simulink model "untitled3"  (R2025b)
settings: Solver=VariableStepAuto  StartTime=0.0  StopTime=10.0  RelTol=1e-3
undefined symbols (not defined in the file): bv, J, K, Kff, Km, Kp, L, R
libraries: slpidlib x8
settings Model: Creator=karadeli  LastModifiedBy=karadeli

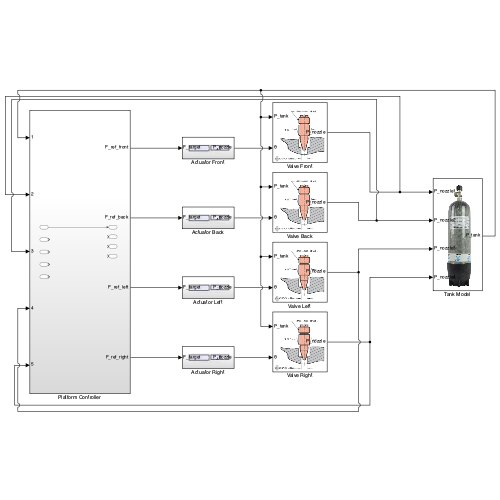
[thumbnail: Simulink's stored preview of the top-level diagram]
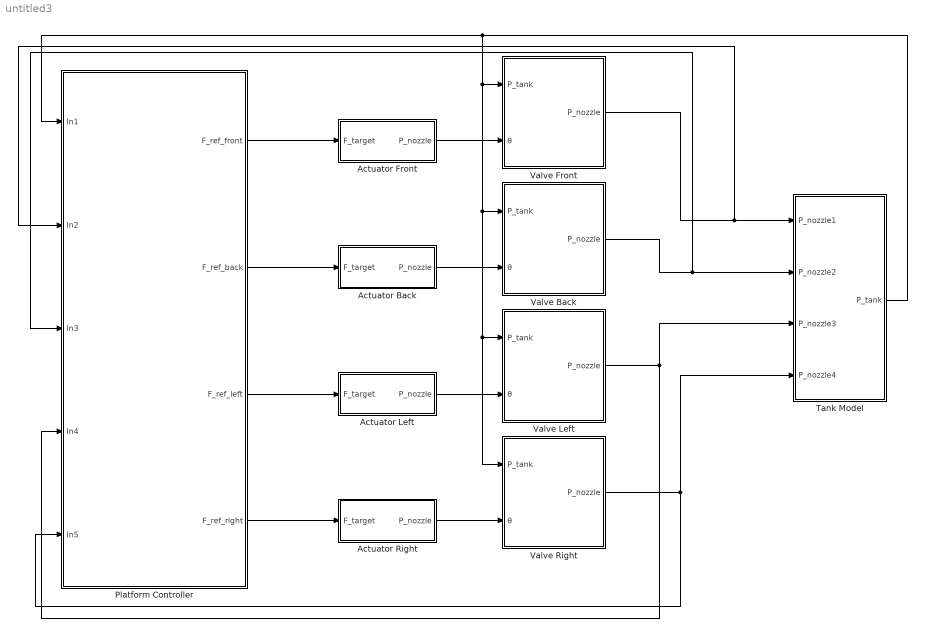
== system untitled3 ==
  Actuator Back : Subsystem
  Actuator Front : Subsystem
  Actuator Left : Subsystem
  Actuator Right : Subsystem
  Platform Controller : Subsystem
  Tank Model : Subsystem
      mask Display: image('Tank.png');
  Valve Back : Subsystem  mask{Parameter1=0}
      mask Display: image('Clippard-Needle-Valves-Overall.png');
  Valve Front : Subsystem  mask{Parameter1=0}
      mask Display: image('Clippard-Needle-Valves-Overall.png');
  Valve Left : Subsystem  mask{Parameter1=0}
      mask Display: image('Clippard-Needle-Valves-Overall.png');
  Valve Right : Subsystem  mask{Parameter1=0}
      mask Display: image('Clippard-Needle-Valves-Overall.png');
  wires:
  Platform Controller/1(F_ref_front) -> Actuator Front/1(F_target)
  Valve Front/1(P_nozzle) -> Platform Controller/2(In2), Tank Model/1(P_nozzle1)
  Tank Model/1(P_tank) -> Valve Right/1(P_tank), Valve Left/1(P_tank), Valve Back/1(P_tank), Valve Front/1(P_tank), Platform Controller/1(In1)
  Valve Back/1(P_nozzle) -> Tank Model/2(P_nozzle2), Platform Controller/3(In3)
  Valve Left/1(P_nozzle) -> Tank Model/3(P_nozzle3), Platform Controller/4(In4)
  Valve Right/1(P_nozzle) -> Tank Model/4(P_nozzle4), Platform Controller/5(In5)
  Actuator Front/1(P_nozzle) -> Valve Front/2(θ)
  Actuator Back/1(P_nozzle) -> Valve Back/2(θ)
  Actuator Left/1(P_nozzle) -> Valve Left/2(θ)
  Actuator Right/1(P_nozzle) -> Valve Right/2(θ)
  Platform Controller/2(F_ref_back) -> Actuator Back/1(F_target)
  Platform Controller/3(F_ref_left) -> Actuator Left/1(F_target)
  Platform Controller/4(F_ref_right) -> Actuator Right/1(F_target)

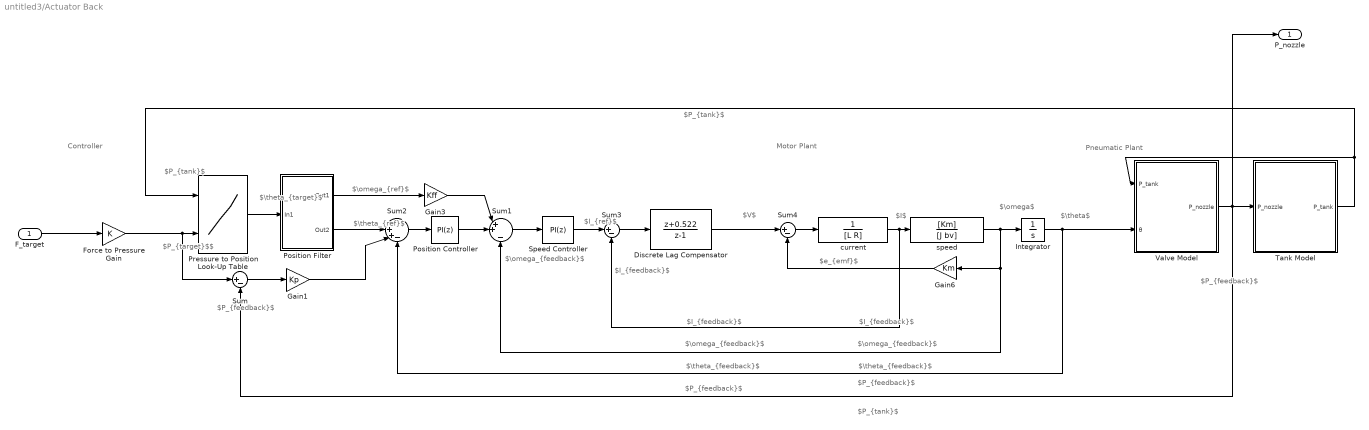
== system untitled3/Actuator Back ==
  note: $P_{tank}$
  note: $\theta_{target}$
  note: Pneumatic Plant
  note: $\theta_{ref}$
  note: $P_{feedback}$
  note: $I_{feedback}$
  note: $I_{ref}$
  note: $\theta_{feedback}$
  note: $e_{emf}$
  note: $P_{feedback}$
  note: $I_{feedback}$
  note: $P_{target}$$
  note: $\theta_{feedback}$
  note: Controller
  note: $P_{feedback}$
  note: $V$
  note: $\omega_{feedback}$
  note: $P_{tank}$
  note: $\omega_{feedback}$
  note: $\omega$
  note: $P_{feedback}$
  note: $I_{feedback}$
  note: $\omega_{feedback}$
  note: $\theta$
  note: Motor Plant
  note: $I$
  note: $P_{tank}$
  note: $\omega_{ref}$
  F_target : Inport
  Discrete Lag Compensator : DiscreteTransferFcn  Numerator=[1 0.522]  Denominator=[1 -1]
  Force to Pressure Gain : Gain  Gain=K
  Gain1 : Gain  Gain=Kp
  Gain3 : Gain  Gain=Kff
  Gain6 : Gain  Gain=Km
  Integrator : Integrator
  Position Controller : slpidlib/PID Controller  Controller=PI  Form=Parallel  TimeDomain=Discrete-time  UseExternalTs=off  SampleTime=-1  IntegratorMethod=Forward Euler  FilterMethod=Forward Euler  ControllerParametersSource=internal  P=1  I=1  UseKiTs=off  D=0  UseExternalDerivativeSource=off  N=100  UseFilter=on  TunerSelectOption=Transfer Function Based (PID Tuner App)  InitialConditionSource=internal  InitialConditionForIntegrator=0  InitialConditionForFilter=0  DifferentiatorICPrevScaledInput=0  ExternalReset=none  TrackingMode=off  Kt=1  LimitOutput=off  SatLimitsSource=internal  UpperSaturationLimit=inf  LowerSaturationLimit=-inf  LinearizeAsGain=on  AntiWindupMode=none  Kb=1  LimitIntegrator=off  UpperIntegratorSaturationLimit=inf  LowerIntegratorSaturationLimit=-inf  POutMin=[]  POutMax=[]  IOutMin=[]  IOutMax=[]  DOutMin=[]  DOutMax=[]  NOutMin=[]  NOutMax=[]  SumOutMin=[]  SumOutMax=[]  SaturationOutMin=[]  SaturationOutMax=[]  PParamMin=[]  PParamMax=[]  IParamMin=[]  IParamMax=[]  DParamMin=[]  DParamMax=[]  NParamMin=[]  NParamMax=[]  KbParamMin=[]  KbParamMax=[]  KtParamMin=[]  KtParamMax=[]  KbOutMin=[]  KbOutMax=[]  KtOutMin=[]  KtOutMax=[]  IntegratorOutMin=[]  IntegratorOutMax=[]  FilterOutMin=[]  FilterOutMax=[]  SumI1OutMin=[]  SumI1OutMax=[]  SumI2OutMin=[]  SumI2OutMax=[]  SumI3OutMin=[]  SumI3OutMax=[]  SumI4OutMin=[]  SumI4OutMax=[]  SumDOutMin=[]  SumDOutMax=[]  DifferentiatorOutMin=[]  DifferentiatorOutMax=[]  FilterDiffOutCoefMin=[]  FilterDiffOutCoefMax=[]  ReciprocalOutMin=[]  ReciprocalOutMax=[]  SumDenOutMin=[]  SumDenOutMax=[]  SumNumOutMin=[]  SumNumOutMax=[]  DivideOutMin=[]  DivideOutMax=[]  UdiffTsProdOutMin=[]  UdiffTsProdOutMax=[]  NTsProdOutMin=[]  NTsProdOutMax=[]  UintegralTsProdOutMin=[]  UintegralTsProdOutMax=[]  UngainTsProdOutMin=[]  UngainTsProdOutMax=[]  ClampingZeroOutDataTypeStr=Inherit: Inherit via back propagation  ClampingZeroOutMin=[]  ClampingZeroOutMax=[]  FilterDenConstantOutDataTypeStr=Inherit: Inherit via back propagation  FilterDenConstantOutMin=[]  FilterDenConstantOutMax=[]  PCopyOutDataTypeStr=Inherit: Inherit via back propagation  PCopyOutMin=[]  PCopyOutMax=[]  NCopyOutDataTypeStr=Inherit: Inherit via back propagation  NCopyOutMin=[]  NCopyOutMax=[]  IntegratorContinuousStateAttributes=''  IntegratorStateMustResolveToSignalObject=off  IntegratorRTWStateStorageClass=Auto  FilterContinuousStateAttributes=''  FilterStateMustResolveToSignalObject=off  FilterRTWStateStorageClass=Auto  ParallelPVariant=InternalParameters  IdealPVariant=Disabled  IVariant=InternalParameters  DVariant=Disabled  IntegratorVariant=Discrete  SatVariant=Disabled  AWVariant=Passthrough  PCopyVariant=Disabled  TRVariant=Disabled  FdbkBlocksVariant=Forward  IdealPFdbkVariant=Disabled  SatFdbkVariant=Disabled  DerivativeFilterVariant=Disabled  NVariant=Disabled  NCopyVariant=Disabled_SignalSpec  FilterICVariant=Disabled  IntegratorICVariant=InternalICs  ExternalResetVariant=Disabled  TRSumVariant=Passthrough  SumFdbkVariant=Disabled  SumVariant=Sum_PI  TsampFilterVariant=InternalTs  TsampNgainVariant=Passthrough  TsampIntegralVariant=Disabled_SignalSpec  ExternalSaturationOutDataTypeStr=Inherit: Same as second input  DerivativeSourceVariant=Disabled  PreIntVariant=InternalPreInt
  Position Filter : Subsystem
      mask Display: dpoly([1], [1/50 1], 's');
  Pressure to Position Look-Up Table : Lookup_n-D  BreakpointsForDimension1=[1:3]  BreakpointsForDimension2=[1:3]  InternalRulePriority=Speed  RndMeth=Simplest
      settings: InputPortMap=u0,u1
  Speed Controller : slpidlib/PID Controller  Controller=PI  Form=Parallel  TimeDomain=Discrete-time  UseExternalTs=off  SampleTime=-1  IntegratorMethod=Forward Euler  FilterMethod=Forward Euler  ControllerParametersSource=internal  P=1  I=1  UseKiTs=off  D=0  UseExternalDerivativeSource=off  N=100  UseFilter=on  TunerSelectOption=Transfer Function Based (PID Tuner App)  InitialConditionSource=internal  InitialConditionForIntegrator=0  InitialConditionForFilter=0  DifferentiatorICPrevScaledInput=0  ExternalReset=none  TrackingMode=off  Kt=1  LimitOutput=off  SatLimitsSource=internal  UpperSaturationLimit=inf  LowerSaturationLimit=-inf  LinearizeAsGain=on  AntiWindupMode=none  Kb=1  LimitIntegrator=off  UpperIntegratorSaturationLimit=inf  LowerIntegratorSaturationLimit=-inf  POutMin=[]  POutMax=[]  IOutMin=[]  IOutMax=[]  DOutMin=[]  DOutMax=[]  NOutMin=[]  NOutMax=[]  SumOutMin=[]  SumOutMax=[]  SaturationOutMin=[]  SaturationOutMax=[]  PParamMin=[]  PParamMax=[]  IParamMin=[]  IParamMax=[]  DParamMin=[]  DParamMax=[]  NParamMin=[]  NParamMax=[]  KbParamMin=[]  KbParamMax=[]  KtParamMin=[]  KtParamMax=[]  KbOutMin=[]  KbOutMax=[]  KtOutMin=[]  KtOutMax=[]  IntegratorOutMin=[]  IntegratorOutMax=[]  FilterOutMin=[]  FilterOutMax=[]  SumI1OutMin=[]  SumI1OutMax=[]  SumI2OutMin=[]  SumI2OutMax=[]  SumI3OutMin=[]  SumI3OutMax=[]  SumI4OutMin=[]  SumI4OutMax=[]  SumDOutMin=[]  SumDOutMax=[]  DifferentiatorOutMin=[]  DifferentiatorOutMax=[]  FilterDiffOutCoefMin=[]  FilterDiffOutCoefMax=[]  ReciprocalOutMin=[]  ReciprocalOutMax=[]  SumDenOutMin=[]  SumDenOutMax=[]  SumNumOutMin=[]  SumNumOutMax=[]  DivideOutMin=[]  DivideOutMax=[]  UdiffTsProdOutMin=[]  UdiffTsProdOutMax=[]  NTsProdOutMin=[]  NTsProdOutMax=[]  UintegralTsProdOutMin=[]  UintegralTsProdOutMax=[]  UngainTsProdOutMin=[]  UngainTsProdOutMax=[]  ClampingZeroOutDataTypeStr=Inherit: Inherit via back propagation  ClampingZeroOutMin=[]  ClampingZeroOutMax=[]  FilterDenConstantOutDataTypeStr=Inherit: Inherit via back propagation  FilterDenConstantOutMin=[]  FilterDenConstantOutMax=[]  PCopyOutDataTypeStr=Inherit: Inherit via back propagation  PCopyOutMin=[]  PCopyOutMax=[]  NCopyOutDataTypeStr=Inherit: Inherit via back propagation  NCopyOutMin=[]  NCopyOutMax=[]  IntegratorContinuousStateAttributes=''  IntegratorStateMustResolveToSignalObject=off  IntegratorRTWStateStorageClass=Auto  FilterContinuousStateAttributes=''  FilterStateMustResolveToSignalObject=off  FilterRTWStateStorageClass=Auto  ParallelPVariant=InternalParameters  IdealPVariant=Disabled  IVariant=InternalParameters  DVariant=Disabled  IntegratorVariant=Discrete  SatVariant=Disabled  AWVariant=Passthrough  PCopyVariant=Disabled  TRVariant=Disabled  FdbkBlocksVariant=Forward  IdealPFdbkVariant=Disabled  SatFdbkVariant=Disabled  DerivativeFilterVariant=Disabled  NVariant=Disabled  NCopyVariant=Disabled_SignalSpec  FilterICVariant=Disabled  IntegratorICVariant=InternalICs  ExternalResetVariant=Disabled  TRSumVariant=Passthrough  SumFdbkVariant=Disabled  SumVariant=Sum_PI  TsampFilterVariant=InternalTs  TsampNgainVariant=Passthrough  TsampIntegralVariant=Disabled_SignalSpec  ExternalSaturationOutDataTypeStr=Inherit: Same as second input  DerivativeSourceVariant=Disabled  PreIntVariant=InternalPreInt
  Sum : Sum  Inputs=|+-
  Sum1 : Sum  Inputs=|++|-
  Sum2 : Sum  Inputs=||++-
  Sum3 : Sum  Inputs=|+-
  Sum4 : Sum  Inputs=|+-
  Tank Model : Subsystem
      mask Display: image('Tank.png');
  Valve Model : Subsystem  mask{Parameter1=0}
      mask Display: image('Clippard-Needle-Valves-Overall.png');
  current : TransferFcn  Denominator=[L R]  ContinuousStateAttributes='current'
  speed : TransferFcn  Numerator=[Km]  Denominator=[J bv]  ContinuousStateAttributes='speed'
  P_nozzle : Outport
  wires:
  speed/1 -> Sum1/3, Gain6/1, Integrator/1
  Tank Model/1(P_tank) -> Pressure to Position Look-Up Table/1, Valve Model/1(P_tank)
  Position Controller/1 -> Sum1/2
  Sum/1 -> Gain1/1
  Pressure to Position Look-Up Table/1 -> Position Filter/1(In1)
  Force to Pressure Gain/1 -> Pressure to Position Look-Up Table/2, Sum/1
  Gain3/1 -> Sum1/1
  F_target/1 -> Force to Pressure Gain/1
  Position Filter/1(Out1) -> Gain3/1
  Sum4/1 -> current/1
  Sum2/1 -> Position Controller/1
  Valve Model/1(P_nozzle) -> Tank Model/1(P_nozzle), P_nozzle/1, Sum/2
  Gain6/1 -> Sum4/2
  Discrete Lag Compensator/1 -> Sum4/1
  Sum3/1 -> Discrete Lag Compensator/1
  Position Filter/2(Out2) -> Sum2/1
  current/1 -> speed/1, Sum3/2
  Speed Controller/1 -> Sum3/1
  Sum1/1 -> Speed Controller/1
  Integrator/1 -> Sum2/3, Valve Model/2(θ)
  Gain1/1 -> Sum2/2

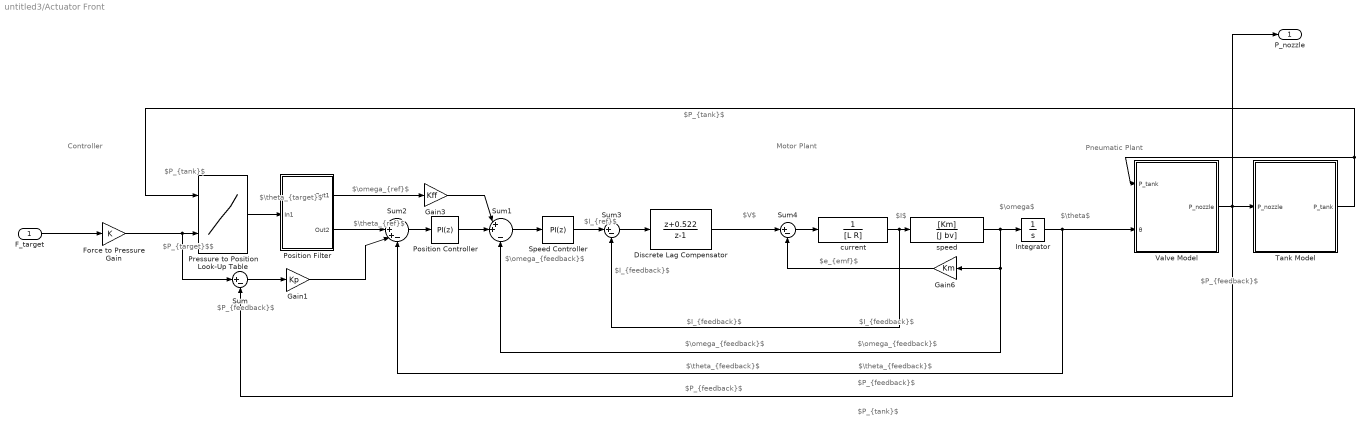
== system untitled3/Actuator Front ==
  note: $\omega_{ref}$
  note: $P_{tank}$
  note: $I$
  note: Motor Plant
  note: $\theta$
  note: $\omega_{feedback}$
  note: $I_{feedback}$
  note: $P_{feedback}$
  note: $\omega$
  note: $\omega_{feedback}$
  note: $P_{tank}$
  note: $\omega_{feedback}$
  note: $V$
  note: $P_{feedback}$
  note: Controller
  note: $\theta_{feedback}$
  note: $P_{target}$$
  note: $I_{feedback}$
  note: $P_{feedback}$
  note: $e_{emf}$
  note: $\theta_{feedback}$
  note: $I_{ref}$
  note: $I_{feedback}$
  note: $P_{feedback}$
  note: $\theta_{ref}$
  note: Pneumatic Plant
  note: $\theta_{target}$
  note: $P_{tank}$
  F_target : Inport
  Discrete Lag Compensator : DiscreteTransferFcn  Numerator=[1 0.522]  Denominator=[1 -1]
  Force to Pressure Gain : Gain  Gain=K
  Gain1 : Gain  Gain=Kp
  Gain3 : Gain  Gain=Kff
  Gain6 : Gain  Gain=Km
  Integrator : Integrator
  Position Controller : slpidlib/PID Controller  Controller=PI  Form=Parallel  TimeDomain=Discrete-time  UseExternalTs=off  SampleTime=-1  IntegratorMethod=Forward Euler  FilterMethod=Forward Euler  ControllerParametersSource=internal  P=1  I=1  UseKiTs=off  D=0  UseExternalDerivativeSource=off  N=100  UseFilter=on  TunerSelectOption=Transfer Function Based (PID Tuner App)  InitialConditionSource=internal  InitialConditionForIntegrator=0  InitialConditionForFilter=0  DifferentiatorICPrevScaledInput=0  ExternalReset=none  TrackingMode=off  Kt=1  LimitOutput=off  SatLimitsSource=internal  UpperSaturationLimit=inf  LowerSaturationLimit=-inf  LinearizeAsGain=on  AntiWindupMode=none  Kb=1  LimitIntegrator=off  UpperIntegratorSaturationLimit=inf  LowerIntegratorSaturationLimit=-inf  POutMin=[]  POutMax=[]  IOutMin=[]  IOutMax=[]  DOutMin=[]  DOutMax=[]  NOutMin=[]  NOutMax=[]  SumOutMin=[]  SumOutMax=[]  SaturationOutMin=[]  SaturationOutMax=[]  PParamMin=[]  PParamMax=[]  IParamMin=[]  IParamMax=[]  DParamMin=[]  DParamMax=[]  NParamMin=[]  NParamMax=[]  KbParamMin=[]  KbParamMax=[]  KtParamMin=[]  KtParamMax=[]  KbOutMin=[]  KbOutMax=[]  KtOutMin=[]  KtOutMax=[]  IntegratorOutMin=[]  IntegratorOutMax=[]  FilterOutMin=[]  FilterOutMax=[]  SumI1OutMin=[]  SumI1OutMax=[]  SumI2OutMin=[]  SumI2OutMax=[]  SumI3OutMin=[]  SumI3OutMax=[]  SumI4OutMin=[]  SumI4OutMax=[]  SumDOutMin=[]  SumDOutMax=[]  DifferentiatorOutMin=[]  DifferentiatorOutMax=[]  FilterDiffOutCoefMin=[]  FilterDiffOutCoefMax=[]  ReciprocalOutMin=[]  ReciprocalOutMax=[]  SumDenOutMin=[]  SumDenOutMax=[]  SumNumOutMin=[]  SumNumOutMax=[]  DivideOutMin=[]  DivideOutMax=[]  UdiffTsProdOutMin=[]  UdiffTsProdOutMax=[]  NTsProdOutMin=[]  NTsProdOutMax=[]  UintegralTsProdOutMin=[]  UintegralTsProdOutMax=[]  UngainTsProdOutMin=[]  UngainTsProdOutMax=[]  ClampingZeroOutDataTypeStr=Inherit: Inherit via back propagation  ClampingZeroOutMin=[]  ClampingZeroOutMax=[]  FilterDenConstantOutDataTypeStr=Inherit: Inherit via back propagation  FilterDenConstantOutMin=[]  FilterDenConstantOutMax=[]  PCopyOutDataTypeStr=Inherit: Inherit via back propagation  PCopyOutMin=[]  PCopyOutMax=[]  NCopyOutDataTypeStr=Inherit: Inherit via back propagation  NCopyOutMin=[]  NCopyOutMax=[]  IntegratorContinuousStateAttributes=''  IntegratorStateMustResolveToSignalObject=off  IntegratorRTWStateStorageClass=Auto  FilterContinuousStateAttributes=''  FilterStateMustResolveToSignalObject=off  FilterRTWStateStorageClass=Auto  ParallelPVariant=InternalParameters  IdealPVariant=Disabled  IVariant=InternalParameters  DVariant=Disabled  IntegratorVariant=Discrete  SatVariant=Disabled  AWVariant=Passthrough  PCopyVariant=Disabled  TRVariant=Disabled  FdbkBlocksVariant=Forward  IdealPFdbkVariant=Disabled  SatFdbkVariant=Disabled  DerivativeFilterVariant=Disabled  NVariant=Disabled  NCopyVariant=Disabled_SignalSpec  FilterICVariant=Disabled  IntegratorICVariant=InternalICs  ExternalResetVariant=Disabled  TRSumVariant=Passthrough  SumFdbkVariant=Disabled  SumVariant=Sum_PI  TsampFilterVariant=InternalTs  TsampNgainVariant=Passthrough  TsampIntegralVariant=Disabled_SignalSpec  ExternalSaturationOutDataTypeStr=Inherit: Same as second input  DerivativeSourceVariant=Disabled  PreIntVariant=InternalPreInt
  Position Filter : Subsystem
      mask Display: dpoly([1], [1/50 1], 's');
  Pressure to Position Look-Up Table : Lookup_n-D  BreakpointsForDimension1=[1:3]  BreakpointsForDimension2=[1:3]  InternalRulePriority=Speed  RndMeth=Simplest
      settings: InputPortMap=u0,u1
  Speed Controller : slpidlib/PID Controller  Controller=PI  Form=Parallel  TimeDomain=Discrete-time  UseExternalTs=off  SampleTime=-1  IntegratorMethod=Forward Euler  FilterMethod=Forward Euler  ControllerParametersSource=internal  P=1  I=1  UseKiTs=off  D=0  UseExternalDerivativeSource=off  N=100  UseFilter=on  TunerSelectOption=Transfer Function Based (PID Tuner App)  InitialConditionSource=internal  InitialConditionForIntegrator=0  InitialConditionForFilter=0  DifferentiatorICPrevScaledInput=0  ExternalReset=none  TrackingMode=off  Kt=1  LimitOutput=off  SatLimitsSource=internal  UpperSaturationLimit=inf  LowerSaturationLimit=-inf  LinearizeAsGain=on  AntiWindupMode=none  Kb=1  LimitIntegrator=off  UpperIntegratorSaturationLimit=inf  LowerIntegratorSaturationLimit=-inf  POutMin=[]  POutMax=[]  IOutMin=[]  IOutMax=[]  DOutMin=[]  DOutMax=[]  NOutMin=[]  NOutMax=[]  SumOutMin=[]  SumOutMax=[]  SaturationOutMin=[]  SaturationOutMax=[]  PParamMin=[]  PParamMax=[]  IParamMin=[]  IParamMax=[]  DParamMin=[]  DParamMax=[]  NParamMin=[]  NParamMax=[]  KbParamMin=[]  KbParamMax=[]  KtParamMin=[]  KtParamMax=[]  KbOutMin=[]  KbOutMax=[]  KtOutMin=[]  KtOutMax=[]  IntegratorOutMin=[]  IntegratorOutMax=[]  FilterOutMin=[]  FilterOutMax=[]  SumI1OutMin=[]  SumI1OutMax=[]  SumI2OutMin=[]  SumI2OutMax=[]  SumI3OutMin=[]  SumI3OutMax=[]  SumI4OutMin=[]  SumI4OutMax=[]  SumDOutMin=[]  SumDOutMax=[]  DifferentiatorOutMin=[]  DifferentiatorOutMax=[]  FilterDiffOutCoefMin=[]  FilterDiffOutCoefMax=[]  ReciprocalOutMin=[]  ReciprocalOutMax=[]  SumDenOutMin=[]  SumDenOutMax=[]  SumNumOutMin=[]  SumNumOutMax=[]  DivideOutMin=[]  DivideOutMax=[]  UdiffTsProdOutMin=[]  UdiffTsProdOutMax=[]  NTsProdOutMin=[]  NTsProdOutMax=[]  UintegralTsProdOutMin=[]  UintegralTsProdOutMax=[]  UngainTsProdOutMin=[]  UngainTsProdOutMax=[]  ClampingZeroOutDataTypeStr=Inherit: Inherit via back propagation  ClampingZeroOutMin=[]  ClampingZeroOutMax=[]  FilterDenConstantOutDataTypeStr=Inherit: Inherit via back propagation  FilterDenConstantOutMin=[]  FilterDenConstantOutMax=[]  PCopyOutDataTypeStr=Inherit: Inherit via back propagation  PCopyOutMin=[]  PCopyOutMax=[]  NCopyOutDataTypeStr=Inherit: Inherit via back propagation  NCopyOutMin=[]  NCopyOutMax=[]  IntegratorContinuousStateAttributes=''  IntegratorStateMustResolveToSignalObject=off  IntegratorRTWStateStorageClass=Auto  FilterContinuousStateAttributes=''  FilterStateMustResolveToSignalObject=off  FilterRTWStateStorageClass=Auto  ParallelPVariant=InternalParameters  IdealPVariant=Disabled  IVariant=InternalParameters  DVariant=Disabled  IntegratorVariant=Discrete  SatVariant=Disabled  AWVariant=Passthrough  PCopyVariant=Disabled  TRVariant=Disabled  FdbkBlocksVariant=Forward  IdealPFdbkVariant=Disabled  SatFdbkVariant=Disabled  DerivativeFilterVariant=Disabled  NVariant=Disabled  NCopyVariant=Disabled_SignalSpec  FilterICVariant=Disabled  IntegratorICVariant=InternalICs  ExternalResetVariant=Disabled  TRSumVariant=Passthrough  SumFdbkVariant=Disabled  SumVariant=Sum_PI  TsampFilterVariant=InternalTs  TsampNgainVariant=Passthrough  TsampIntegralVariant=Disabled_SignalSpec  ExternalSaturationOutDataTypeStr=Inherit: Same as second input  DerivativeSourceVariant=Disabled  PreIntVariant=InternalPreInt
  Sum : Sum  Inputs=|+-
  Sum1 : Sum  Inputs=|++|-
  Sum2 : Sum  Inputs=||++-
  Sum3 : Sum  Inputs=|+-
  Sum4 : Sum  Inputs=|+-
  Tank Model : Subsystem
      mask Display: image('Tank.png');
  Valve Model : Subsystem  mask{Parameter1=0}
      mask Display: image('Clippard-Needle-Valves-Overall.png');
  current : TransferFcn  Denominator=[L R]  ContinuousStateAttributes='current'
  speed : TransferFcn  Numerator=[Km]  Denominator=[J bv]  ContinuousStateAttributes='speed'
  P_nozzle : Outport
  wires:
  Gain1/1 -> Sum2/2
  Integrator/1 -> Valve Model/2(θ), Sum2/3
  Sum1/1 -> Speed Controller/1
  Speed Controller/1 -> Sum3/1
  current/1 -> Sum3/2, speed/1
  Position Filter/2(Out2) -> Sum2/1
  Sum3/1 -> Discrete Lag Compensator/1
  Discrete Lag Compensator/1 -> Sum4/1
  Gain6/1 -> Sum4/2
  Valve Model/1(P_nozzle) -> Sum/2, P_nozzle/1, Tank Model/1(P_nozzle)
  Sum2/1 -> Position Controller/1
  Sum4/1 -> current/1
  Position Filter/1(Out1) -> Gain3/1
  F_target/1 -> Force to Pressure Gain/1
  Gain3/1 -> Sum1/1
  Force to Pressure Gain/1 -> Sum/1, Pressure to Position Look-Up Table/2
  Pressure to Position Look-Up Table/1 -> Position Filter/1(In1)
  Sum/1 -> Gain1/1
  Position Controller/1 -> Sum1/2
  Tank Model/1(P_tank) -> Valve Model/1(P_tank), Pressure to Position Look-Up Table/1
  speed/1 -> Integrator/1, Gain6/1, Sum1/3

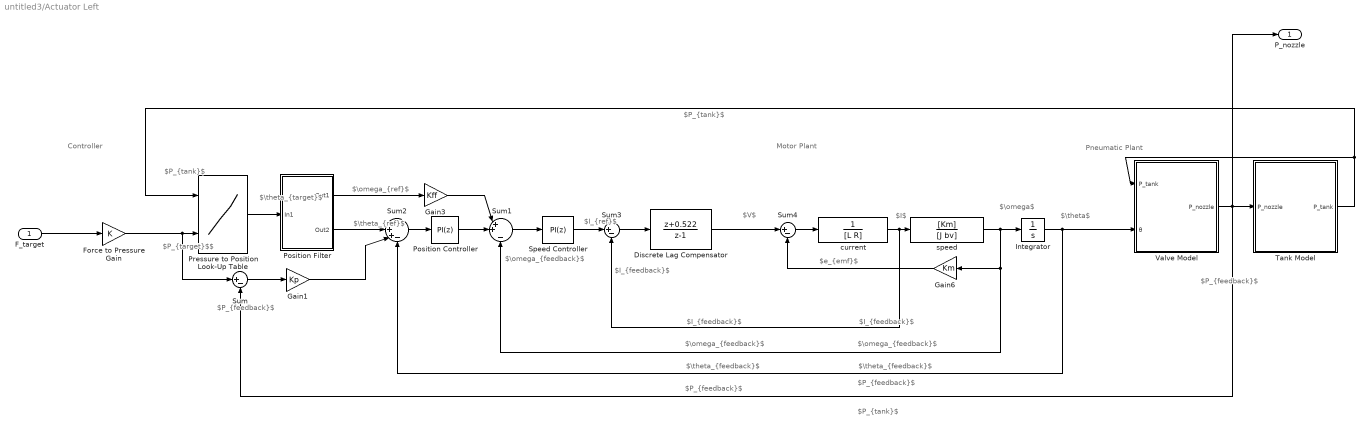
== system untitled3/Actuator Left ==
  note: $\omega_{ref}$
  note: $P_{tank}$
  note: $I$
  note: Motor Plant
  note: $\theta$
  note: $\omega_{feedback}$
  note: $I_{feedback}$
  note: $P_{feedback}$
  note: $\omega$
  note: $\omega_{feedback}$
  note: $P_{tank}$
  note: $\omega_{feedback}$
  note: $V$
  note: $P_{feedback}$
  note: Controller
  note: $\theta_{feedback}$
  note: $P_{target}$$
  note: $I_{feedback}$
  note: $P_{feedback}$
  note: $e_{emf}$
  note: $\theta_{feedback}$
  note: $I_{ref}$
  note: $I_{feedback}$
  note: $P_{feedback}$
  note: $\theta_{ref}$
  note: Pneumatic Plant
  note: $\theta_{target}$
  note: $P_{tank}$
  F_target : Inport
  Discrete Lag Compensator : DiscreteTransferFcn  Numerator=[1 0.522]  Denominator=[1 -1]
  Force to Pressure Gain : Gain  Gain=K
  Gain1 : Gain  Gain=Kp
  Gain3 : Gain  Gain=Kff
  Gain6 : Gain  Gain=Km
  Integrator : Integrator
  Position Controller : slpidlib/PID Controller  Controller=PI  Form=Parallel  TimeDomain=Discrete-time  UseExternalTs=off  SampleTime=-1  IntegratorMethod=Forward Euler  FilterMethod=Forward Euler  ControllerParametersSource=internal  P=1  I=1  UseKiTs=off  D=0  UseExternalDerivativeSource=off  N=100  UseFilter=on  TunerSelectOption=Transfer Function Based (PID Tuner App)  InitialConditionSource=internal  InitialConditionForIntegrator=0  InitialConditionForFilter=0  DifferentiatorICPrevScaledInput=0  ExternalReset=none  TrackingMode=off  Kt=1  LimitOutput=off  SatLimitsSource=internal  UpperSaturationLimit=inf  LowerSaturationLimit=-inf  LinearizeAsGain=on  AntiWindupMode=none  Kb=1  LimitIntegrator=off  UpperIntegratorSaturationLimit=inf  LowerIntegratorSaturationLimit=-inf  POutMin=[]  POutMax=[]  IOutMin=[]  IOutMax=[]  DOutMin=[]  DOutMax=[]  NOutMin=[]  NOutMax=[]  SumOutMin=[]  SumOutMax=[]  SaturationOutMin=[]  SaturationOutMax=[]  PParamMin=[]  PParamMax=[]  IParamMin=[]  IParamMax=[]  DParamMin=[]  DParamMax=[]  NParamMin=[]  NParamMax=[]  KbParamMin=[]  KbParamMax=[]  KtParamMin=[]  KtParamMax=[]  KbOutMin=[]  KbOutMax=[]  KtOutMin=[]  KtOutMax=[]  IntegratorOutMin=[]  IntegratorOutMax=[]  FilterOutMin=[]  FilterOutMax=[]  SumI1OutMin=[]  SumI1OutMax=[]  SumI2OutMin=[]  SumI2OutMax=[]  SumI3OutMin=[]  SumI3OutMax=[]  SumI4OutMin=[]  SumI4OutMax=[]  SumDOutMin=[]  SumDOutMax=[]  DifferentiatorOutMin=[]  DifferentiatorOutMax=[]  FilterDiffOutCoefMin=[]  FilterDiffOutCoefMax=[]  ReciprocalOutMin=[]  ReciprocalOutMax=[]  SumDenOutMin=[]  SumDenOutMax=[]  SumNumOutMin=[]  SumNumOutMax=[]  DivideOutMin=[]  DivideOutMax=[]  UdiffTsProdOutMin=[]  UdiffTsProdOutMax=[]  NTsProdOutMin=[]  NTsProdOutMax=[]  UintegralTsProdOutMin=[]  UintegralTsProdOutMax=[]  UngainTsProdOutMin=[]  UngainTsProdOutMax=[]  ClampingZeroOutDataTypeStr=Inherit: Inherit via back propagation  ClampingZeroOutMin=[]  ClampingZeroOutMax=[]  FilterDenConstantOutDataTypeStr=Inherit: Inherit via back propagation  FilterDenConstantOutMin=[]  FilterDenConstantOutMax=[]  PCopyOutDataTypeStr=Inherit: Inherit via back propagation  PCopyOutMin=[]  PCopyOutMax=[]  NCopyOutDataTypeStr=Inherit: Inherit via back propagation  NCopyOutMin=[]  NCopyOutMax=[]  IntegratorContinuousStateAttributes=''  IntegratorStateMustResolveToSignalObject=off  IntegratorRTWStateStorageClass=Auto  FilterContinuousStateAttributes=''  FilterStateMustResolveToSignalObject=off  FilterRTWStateStorageClass=Auto  ParallelPVariant=InternalParameters  IdealPVariant=Disabled  IVariant=InternalParameters  DVariant=Disabled  IntegratorVariant=Discrete  SatVariant=Disabled  AWVariant=Passthrough  PCopyVariant=Disabled  TRVariant=Disabled  FdbkBlocksVariant=Forward  IdealPFdbkVariant=Disabled  SatFdbkVariant=Disabled  DerivativeFilterVariant=Disabled  NVariant=Disabled  NCopyVariant=Disabled_SignalSpec  FilterICVariant=Disabled  IntegratorICVariant=InternalICs  ExternalResetVariant=Disabled  TRSumVariant=Passthrough  SumFdbkVariant=Disabled  SumVariant=Sum_PI  TsampFilterVariant=InternalTs  TsampNgainVariant=Passthrough  TsampIntegralVariant=Disabled_SignalSpec  ExternalSaturationOutDataTypeStr=Inherit: Same as second input  DerivativeSourceVariant=Disabled  PreIntVariant=InternalPreInt
  Position Filter : Subsystem
      mask Display: dpoly([1], [1/50 1], 's');
  Pressure to Position Look-Up Table : Lookup_n-D  BreakpointsForDimension1=[1:3]  BreakpointsForDimension2=[1:3]  InternalRulePriority=Speed  RndMeth=Simplest
      settings: InputPortMap=u0,u1
  Speed Controller : slpidlib/PID Controller  Controller=PI  Form=Parallel  TimeDomain=Discrete-time  UseExternalTs=off  SampleTime=-1  IntegratorMethod=Forward Euler  FilterMethod=Forward Euler  ControllerParametersSource=internal  P=1  I=1  UseKiTs=off  D=0  UseExternalDerivativeSource=off  N=100  UseFilter=on  TunerSelectOption=Transfer Function Based (PID Tuner App)  InitialConditionSource=internal  InitialConditionForIntegrator=0  InitialConditionForFilter=0  DifferentiatorICPrevScaledInput=0  ExternalReset=none  TrackingMode=off  Kt=1  LimitOutput=off  SatLimitsSource=internal  UpperSaturationLimit=inf  LowerSaturationLimit=-inf  LinearizeAsGain=on  AntiWindupMode=none  Kb=1  LimitIntegrator=off  UpperIntegratorSaturationLimit=inf  LowerIntegratorSaturationLimit=-inf  POutMin=[]  POutMax=[]  IOutMin=[]  IOutMax=[]  DOutMin=[]  DOutMax=[]  NOutMin=[]  NOutMax=[]  SumOutMin=[]  SumOutMax=[]  SaturationOutMin=[]  SaturationOutMax=[]  PParamMin=[]  PParamMax=[]  IParamMin=[]  IParamMax=[]  DParamMin=[]  DParamMax=[]  NParamMin=[]  NParamMax=[]  KbParamMin=[]  KbParamMax=[]  KtParamMin=[]  KtParamMax=[]  KbOutMin=[]  KbOutMax=[]  KtOutMin=[]  KtOutMax=[]  IntegratorOutMin=[]  IntegratorOutMax=[]  FilterOutMin=[]  FilterOutMax=[]  SumI1OutMin=[]  SumI1OutMax=[]  SumI2OutMin=[]  SumI2OutMax=[]  SumI3OutMin=[]  SumI3OutMax=[]  SumI4OutMin=[]  SumI4OutMax=[]  SumDOutMin=[]  SumDOutMax=[]  DifferentiatorOutMin=[]  DifferentiatorOutMax=[]  FilterDiffOutCoefMin=[]  FilterDiffOutCoefMax=[]  ReciprocalOutMin=[]  ReciprocalOutMax=[]  SumDenOutMin=[]  SumDenOutMax=[]  SumNumOutMin=[]  SumNumOutMax=[]  DivideOutMin=[]  DivideOutMax=[]  UdiffTsProdOutMin=[]  UdiffTsProdOutMax=[]  NTsProdOutMin=[]  NTsProdOutMax=[]  UintegralTsProdOutMin=[]  UintegralTsProdOutMax=[]  UngainTsProdOutMin=[]  UngainTsProdOutMax=[]  ClampingZeroOutDataTypeStr=Inherit: Inherit via back propagation  ClampingZeroOutMin=[]  ClampingZeroOutMax=[]  FilterDenConstantOutDataTypeStr=Inherit: Inherit via back propagation  FilterDenConstantOutMin=[]  FilterDenConstantOutMax=[]  PCopyOutDataTypeStr=Inherit: Inherit via back propagation  PCopyOutMin=[]  PCopyOutMax=[]  NCopyOutDataTypeStr=Inherit: Inherit via back propagation  NCopyOutMin=[]  NCopyOutMax=[]  IntegratorContinuousStateAttributes=''  IntegratorStateMustResolveToSignalObject=off  IntegratorRTWStateStorageClass=Auto  FilterContinuousStateAttributes=''  FilterStateMustResolveToSignalObject=off  FilterRTWStateStorageClass=Auto  ParallelPVariant=InternalParameters  IdealPVariant=Disabled  IVariant=InternalParameters  DVariant=Disabled  IntegratorVariant=Discrete  SatVariant=Disabled  AWVariant=Passthrough  PCopyVariant=Disabled  TRVariant=Disabled  FdbkBlocksVariant=Forward  IdealPFdbkVariant=Disabled  SatFdbkVariant=Disabled  DerivativeFilterVariant=Disabled  NVariant=Disabled  NCopyVariant=Disabled_SignalSpec  FilterICVariant=Disabled  IntegratorICVariant=InternalICs  ExternalResetVariant=Disabled  TRSumVariant=Passthrough  SumFdbkVariant=Disabled  SumVariant=Sum_PI  TsampFilterVariant=InternalTs  TsampNgainVariant=Passthrough  TsampIntegralVariant=Disabled_SignalSpec  ExternalSaturationOutDataTypeStr=Inherit: Same as second input  DerivativeSourceVariant=Disabled  PreIntVariant=InternalPreInt
  Sum : Sum  Inputs=|+-
  Sum1 : Sum  Inputs=|++|-
  Sum2 : Sum  Inputs=||++-
  Sum3 : Sum  Inputs=|+-
  Sum4 : Sum  Inputs=|+-
  Tank Model : Subsystem
      mask Display: image('Tank.png');
  Valve Model : Subsystem  mask{Parameter1=0}
      mask Display: image('Clippard-Needle-Valves-Overall.png');
  current : TransferFcn  Denominator=[L R]  ContinuousStateAttributes='current'
  speed : TransferFcn  Numerator=[Km]  Denominator=[J bv]  ContinuousStateAttributes='speed'
  P_nozzle : Outport
  wires:
  Gain1/1 -> Sum2/2
  Integrator/1 -> Valve Model/2(θ), Sum2/3
  Sum1/1 -> Speed Controller/1
  Speed Controller/1 -> Sum3/1
  current/1 -> Sum3/2, speed/1
  Position Filter/2(Out2) -> Sum2/1
  Sum3/1 -> Discrete Lag Compensator/1
  Discrete Lag Compensator/1 -> Sum4/1
  Gain6/1 -> Sum4/2
  Valve Model/1(P_nozzle) -> Sum/2, P_nozzle/1, Tank Model/1(P_nozzle)
  Sum2/1 -> Position Controller/1
  Sum4/1 -> current/1
  Position Filter/1(Out1) -> Gain3/1
  F_target/1 -> Force to Pressure Gain/1
  Gain3/1 -> Sum1/1
  Force to Pressure Gain/1 -> Sum/1, Pressure to Position Look-Up Table/2
  Pressure to Position Look-Up Table/1 -> Position Filter/1(In1)
  Sum/1 -> Gain1/1
  Position Controller/1 -> Sum1/2
  Tank Model/1(P_tank) -> Valve Model/1(P_tank), Pressure to Position Look-Up Table/1
  speed/1 -> Integrator/1, Gain6/1, Sum1/3

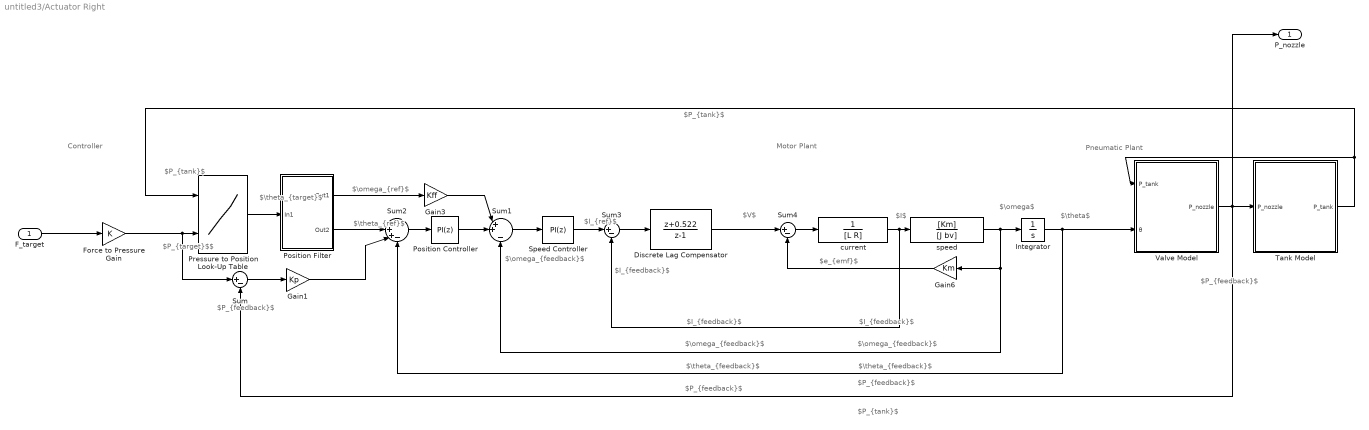
== system untitled3/Actuator Right ==
  note: $P_{tank}$
  note: $\theta_{target}$
  note: Pneumatic Plant
  note: $\theta_{ref}$
  note: $P_{feedback}$
  note: $I_{feedback}$
  note: $I_{ref}$
  note: $\theta_{feedback}$
  note: $e_{emf}$
  note: $P_{feedback}$
  note: $I_{feedback}$
  note: $P_{target}$$
  note: $\theta_{feedback}$
  note: Controller
  note: $P_{feedback}$
  note: $V$
  note: $\omega_{feedback}$
  note: $P_{tank}$
  note: $\omega_{feedback}$
  note: $\omega$
  note: $P_{feedback}$
  note: $I_{feedback}$
  note: $\omega_{feedback}$
  note: $\theta$
  note: Motor Plant
  note: $I$
  note: $P_{tank}$
  note: $\omega_{ref}$
  F_target : Inport
  Discrete Lag Compensator : DiscreteTransferFcn  Numerator=[1 0.522]  Denominator=[1 -1]
  Force to Pressure Gain : Gain  Gain=K
  Gain1 : Gain  Gain=Kp
  Gain3 : Gain  Gain=Kff
  Gain6 : Gain  Gain=Km
  Integrator : Integrator
  Position Controller : slpidlib/PID Controller  Controller=PI  Form=Parallel  TimeDomain=Discrete-time  UseExternalTs=off  SampleTime=-1  IntegratorMethod=Forward Euler  FilterMethod=Forward Euler  ControllerParametersSource=internal  P=1  I=1  UseKiTs=off  D=0  UseExternalDerivativeSource=off  N=100  UseFilter=on  TunerSelectOption=Transfer Function Based (PID Tuner App)  InitialConditionSource=internal  InitialConditionForIntegrator=0  InitialConditionForFilter=0  DifferentiatorICPrevScaledInput=0  ExternalReset=none  TrackingMode=off  Kt=1  LimitOutput=off  SatLimitsSource=internal  UpperSaturationLimit=inf  LowerSaturationLimit=-inf  LinearizeAsGain=on  AntiWindupMode=none  Kb=1  LimitIntegrator=off  UpperIntegratorSaturationLimit=inf  LowerIntegratorSaturationLimit=-inf  POutMin=[]  POutMax=[]  IOutMin=[]  IOutMax=[]  DOutMin=[]  DOutMax=[]  NOutMin=[]  NOutMax=[]  SumOutMin=[]  SumOutMax=[]  SaturationOutMin=[]  SaturationOutMax=[]  PParamMin=[]  PParamMax=[]  IParamMin=[]  IParamMax=[]  DParamMin=[]  DParamMax=[]  NParamMin=[]  NParamMax=[]  KbParamMin=[]  KbParamMax=[]  KtParamMin=[]  KtParamMax=[]  KbOutMin=[]  KbOutMax=[]  KtOutMin=[]  KtOutMax=[]  IntegratorOutMin=[]  IntegratorOutMax=[]  FilterOutMin=[]  FilterOutMax=[]  SumI1OutMin=[]  SumI1OutMax=[]  SumI2OutMin=[]  SumI2OutMax=[]  SumI3OutMin=[]  SumI3OutMax=[]  SumI4OutMin=[]  SumI4OutMax=[]  SumDOutMin=[]  SumDOutMax=[]  DifferentiatorOutMin=[]  DifferentiatorOutMax=[]  FilterDiffOutCoefMin=[]  FilterDiffOutCoefMax=[]  ReciprocalOutMin=[]  ReciprocalOutMax=[]  SumDenOutMin=[]  SumDenOutMax=[]  SumNumOutMin=[]  SumNumOutMax=[]  DivideOutMin=[]  DivideOutMax=[]  UdiffTsProdOutMin=[]  UdiffTsProdOutMax=[]  NTsProdOutMin=[]  NTsProdOutMax=[]  UintegralTsProdOutMin=[]  UintegralTsProdOutMax=[]  UngainTsProdOutMin=[]  UngainTsProdOutMax=[]  ClampingZeroOutDataTypeStr=Inherit: Inherit via back propagation  ClampingZeroOutMin=[]  ClampingZeroOutMax=[]  FilterDenConstantOutDataTypeStr=Inherit: Inherit via back propagation  FilterDenConstantOutMin=[]  FilterDenConstantOutMax=[]  PCopyOutDataTypeStr=Inherit: Inherit via back propagation  PCopyOutMin=[]  PCopyOutMax=[]  NCopyOutDataTypeStr=Inherit: Inherit via back propagation  NCopyOutMin=[]  NCopyOutMax=[]  IntegratorContinuousStateAttributes=''  IntegratorStateMustResolveToSignalObject=off  IntegratorRTWStateStorageClass=Auto  FilterContinuousStateAttributes=''  FilterStateMustResolveToSignalObject=off  FilterRTWStateStorageClass=Auto  ParallelPVariant=InternalParameters  IdealPVariant=Disabled  IVariant=InternalParameters  DVariant=Disabled  IntegratorVariant=Discrete  SatVariant=Disabled  AWVariant=Passthrough  PCopyVariant=Disabled  TRVariant=Disabled  FdbkBlocksVariant=Forward  IdealPFdbkVariant=Disabled  SatFdbkVariant=Disabled  DerivativeFilterVariant=Disabled  NVariant=Disabled  NCopyVariant=Disabled_SignalSpec  FilterICVariant=Disabled  IntegratorICVariant=InternalICs  ExternalResetVariant=Disabled  TRSumVariant=Passthrough  SumFdbkVariant=Disabled  SumVariant=Sum_PI  TsampFilterVariant=InternalTs  TsampNgainVariant=Passthrough  TsampIntegralVariant=Disabled_SignalSpec  ExternalSaturationOutDataTypeStr=Inherit: Same as second input  DerivativeSourceVariant=Disabled  PreIntVariant=InternalPreInt
  Position Filter : Subsystem
      mask Display: dpoly([1], [1/50 1], 's');
  Pressure to Position Look-Up Table : Lookup_n-D  BreakpointsForDimension1=[1:3]  BreakpointsForDimension2=[1:3]  InternalRulePriority=Speed  RndMeth=Simplest
      settings: InputPortMap=u0,u1
  Speed Controller : slpidlib/PID Controller  Controller=PI  Form=Parallel  TimeDomain=Discrete-time  UseExternalTs=off  SampleTime=-1  IntegratorMethod=Forward Euler  FilterMethod=Forward Euler  ControllerParametersSource=internal  P=1  I=1  UseKiTs=off  D=0  UseExternalDerivativeSource=off  N=100  UseFilter=on  TunerSelectOption=Transfer Function Based (PID Tuner App)  InitialConditionSource=internal  InitialConditionForIntegrator=0  InitialConditionForFilter=0  DifferentiatorICPrevScaledInput=0  ExternalReset=none  TrackingMode=off  Kt=1  LimitOutput=off  SatLimitsSource=internal  UpperSaturationLimit=inf  LowerSaturationLimit=-inf  LinearizeAsGain=on  AntiWindupMode=none  Kb=1  LimitIntegrator=off  UpperIntegratorSaturationLimit=inf  LowerIntegratorSaturationLimit=-inf  POutMin=[]  POutMax=[]  IOutMin=[]  IOutMax=[]  DOutMin=[]  DOutMax=[]  NOutMin=[]  NOutMax=[]  SumOutMin=[]  SumOutMax=[]  SaturationOutMin=[]  SaturationOutMax=[]  PParamMin=[]  PParamMax=[]  IParamMin=[]  IParamMax=[]  DParamMin=[]  DParamMax=[]  NParamMin=[]  NParamMax=[]  KbParamMin=[]  KbParamMax=[]  KtParamMin=[]  KtParamMax=[]  KbOutMin=[]  KbOutMax=[]  KtOutMin=[]  KtOutMax=[]  IntegratorOutMin=[]  IntegratorOutMax=[]  FilterOutMin=[]  FilterOutMax=[]  SumI1OutMin=[]  SumI1OutMax=[]  SumI2OutMin=[]  SumI2OutMax=[]  SumI3OutMin=[]  SumI3OutMax=[]  SumI4OutMin=[]  SumI4OutMax=[]  SumDOutMin=[]  SumDOutMax=[]  DifferentiatorOutMin=[]  DifferentiatorOutMax=[]  FilterDiffOutCoefMin=[]  FilterDiffOutCoefMax=[]  ReciprocalOutMin=[]  ReciprocalOutMax=[]  SumDenOutMin=[]  SumDenOutMax=[]  SumNumOutMin=[]  SumNumOutMax=[]  DivideOutMin=[]  DivideOutMax=[]  UdiffTsProdOutMin=[]  UdiffTsProdOutMax=[]  NTsProdOutMin=[]  NTsProdOutMax=[]  UintegralTsProdOutMin=[]  UintegralTsProdOutMax=[]  UngainTsProdOutMin=[]  UngainTsProdOutMax=[]  ClampingZeroOutDataTypeStr=Inherit: Inherit via back propagation  ClampingZeroOutMin=[]  ClampingZeroOutMax=[]  FilterDenConstantOutDataTypeStr=Inherit: Inherit via back propagation  FilterDenConstantOutMin=[]  FilterDenConstantOutMax=[]  PCopyOutDataTypeStr=Inherit: Inherit via back propagation  PCopyOutMin=[]  PCopyOutMax=[]  NCopyOutDataTypeStr=Inherit: Inherit via back propagation  NCopyOutMin=[]  NCopyOutMax=[]  IntegratorContinuousStateAttributes=''  IntegratorStateMustResolveToSignalObject=off  IntegratorRTWStateStorageClass=Auto  FilterContinuousStateAttributes=''  FilterStateMustResolveToSignalObject=off  FilterRTWStateStorageClass=Auto  ParallelPVariant=InternalParameters  IdealPVariant=Disabled  IVariant=InternalParameters  DVariant=Disabled  IntegratorVariant=Discrete  SatVariant=Disabled  AWVariant=Passthrough  PCopyVariant=Disabled  TRVariant=Disabled  FdbkBlocksVariant=Forward  IdealPFdbkVariant=Disabled  SatFdbkVariant=Disabled  DerivativeFilterVariant=Disabled  NVariant=Disabled  NCopyVariant=Disabled_SignalSpec  FilterICVariant=Disabled  IntegratorICVariant=InternalICs  ExternalResetVariant=Disabled  TRSumVariant=Passthrough  SumFdbkVariant=Disabled  SumVariant=Sum_PI  TsampFilterVariant=InternalTs  TsampNgainVariant=Passthrough  TsampIntegralVariant=Disabled_SignalSpec  ExternalSaturationOutDataTypeStr=Inherit: Same as second input  DerivativeSourceVariant=Disabled  PreIntVariant=InternalPreInt
  Sum : Sum  Inputs=|+-
  Sum1 : Sum  Inputs=|++|-
  Sum2 : Sum  Inputs=||++-
  Sum3 : Sum  Inputs=|+-
  Sum4 : Sum  Inputs=|+-
  Tank Model : Subsystem
      mask Display: image('Tank.png');
  Valve Model : Subsystem  mask{Parameter1=0}
      mask Display: image('Clippard-Needle-Valves-Overall.png');
  current : TransferFcn  Denominator=[L R]  ContinuousStateAttributes='current'
  speed : TransferFcn  Numerator=[Km]  Denominator=[J bv]  ContinuousStateAttributes='speed'
  P_nozzle : Outport
  wires:
  speed/1 -> Sum1/3, Gain6/1, Integrator/1
  Tank Model/1(P_tank) -> Pressure to Position Look-Up Table/1, Valve Model/1(P_tank)
  Position Controller/1 -> Sum1/2
  Sum/1 -> Gain1/1
  Pressure to Position Look-Up Table/1 -> Position Filter/1(In1)
  Force to Pressure Gain/1 -> Pressure to Position Look-Up Table/2, Sum/1
  Gain3/1 -> Sum1/1
  F_target/1 -> Force to Pressure Gain/1
  Position Filter/1(Out1) -> Gain3/1
  Sum4/1 -> current/1
  Sum2/1 -> Position Controller/1
  Valve Model/1(P_nozzle) -> Tank Model/1(P_nozzle), P_nozzle/1, Sum/2
  Gain6/1 -> Sum4/2
  Discrete Lag Compensator/1 -> Sum4/1
  Sum3/1 -> Discrete Lag Compensator/1
  Position Filter/2(Out2) -> Sum2/1
  current/1 -> speed/1, Sum3/2
  Speed Controller/1 -> Sum3/1
  Sum1/1 -> Speed Controller/1
  Integrator/1 -> Sum2/3, Valve Model/2(θ)
  Gain1/1 -> Sum2/2

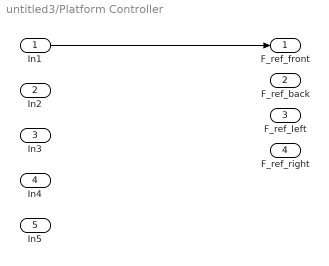
== system untitled3/Platform Controller ==
  In1 : Inport
  In2 : Inport  Port=2
  In3 : Inport  Port=3
  In4 : Inport  Port=4
  In5 : Inport  Port=5
  F_ref_front : Outport
  F_ref_back : Outport  Port=2
  F_ref_left : Outport  Port=3
  F_ref_right : Outport  Port=4
  wires:
  In1/1 -> F_ref_front/1

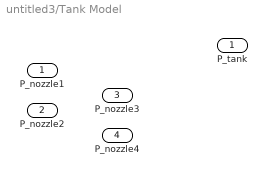
== system untitled3/Tank Model ==
  P_nozzle1 : Inport
  P_nozzle2 : Inport  Port=2
  P_nozzle3 : Inport  Port=3
  P_nozzle4 : Inport  Port=4
  P_tank : Outport

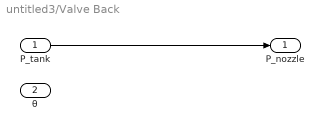
== system untitled3/Valve Back ==
  P_tank : Inport
  θ : Inport  Port=2
  P_nozzle : Outport
  wires:
  P_tank/1 -> P_nozzle/1

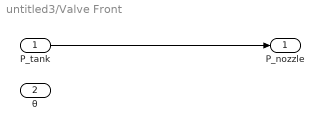
== system untitled3/Valve Front ==
  P_tank : Inport
  θ : Inport  Port=2
  P_nozzle : Outport
  wires:
  P_tank/1 -> P_nozzle/1

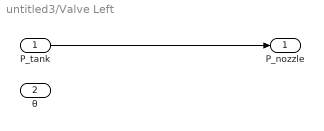
== system untitled3/Valve Left ==
  P_tank : Inport
  θ : Inport  Port=2
  P_nozzle : Outport
  wires:
  P_tank/1 -> P_nozzle/1

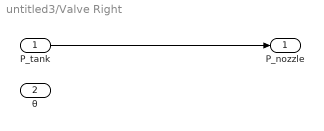
== system untitled3/Valve Right ==
  P_tank : Inport
  θ : Inport  Port=2
  P_nozzle : Outport
  wires:
  P_tank/1 -> P_nozzle/1

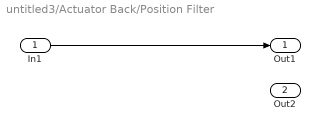
== system untitled3/Actuator Back/Position Filter ==
  In1 : Inport
  Out1 : Outport
  Out2 : Outport  Port=2
  wires:
  In1/1 -> Out1/1

== system untitled3/Actuator Back/Tank Model ==
  P_nozzle : Inport
  P_tank : Outport

== system untitled3/Actuator Back/Valve Model ==
  P_tank : Inport
  θ : Inport  Port=2
  P_nozzle : Outport
  wires:
  P_tank/1 -> P_nozzle/1

== system untitled3/Actuator Front/Position Filter ==
  In1 : Inport
  Out1 : Outport
  Out2 : Outport  Port=2
  wires:
  In1/1 -> Out1/1

== system untitled3/Actuator Front/Tank Model ==
  P_nozzle : Inport
  P_tank : Outport

== system untitled3/Actuator Front/Valve Model ==
  P_tank : Inport
  θ : Inport  Port=2
  P_nozzle : Outport
  wires:
  P_tank/1 -> P_nozzle/1

== system untitled3/Actuator Left/Position Filter ==
  In1 : Inport
  Out1 : Outport
  Out2 : Outport  Port=2
  wires:
  In1/1 -> Out1/1

== system untitled3/Actuator Left/Tank Model ==
  P_nozzle : Inport
  P_tank : Outport

== system untitled3/Actuator Left/Valve Model ==
  P_tank : Inport
  θ : Inport  Port=2
  P_nozzle : Outport
  wires:
  P_tank/1 -> P_nozzle/1

== system untitled3/Actuator Right/Position Filter ==
  In1 : Inport
  Out1 : Outport
  Out2 : Outport  Port=2
  wires:
  In1/1 -> Out1/1

== system untitled3/Actuator Right/Tank Model ==
  P_nozzle : Inport
  P_tank : Outport

== system untitled3/Actuator Right/Valve Model ==
  P_tank : Inport
  θ : Inport  Port=2
  P_nozzle : Outport
  wires:
  P_tank/1 -> P_nozzle/1
